simulink model "no1"  (R2024a)
settings: Solver=VariableStepAuto  StartTime=0.0  StopTime=20.0  RelTol=1e-3
values from neighbouring files (symbols this model uses):
  G1_den = [1 0 0]    [BLOCK DIAGRAM NO.1.m]    (also in MALABANAN_MALIBIRAN_NO2_CODE.m; NO1.m)
  G1_num = [0 0 1]    [BLOCK DIAGRAM NO.1.m]    (also in MALABANAN_MALIBIRAN_NO2_CODE.m = [0 1]; NO1.m)
  G2_den = [1 1]    [BLOCK DIAGRAM NO.1.m]    (also in MALABANAN_MALIBIRAN_NO2_CODE.m; NO1.m)
  G2_num = [0 1]    [BLOCK DIAGRAM NO.1.m]    (also in MALABANAN_MALIBIRAN_NO2_CODE.m; NO1.m)
  G2_num_num = [1 2]    [BLOCK DIAGRAM NO.1.m]    (also in NO1.m)
  G2_sum_den = conv(G2_den, G2_num)    [BLOCK DIAGRAM NO.1.m]    (also in NO1.m)
  G3_den = [1 0]    [BLOCK DIAGRAM NO.1.m]    (also in MALABANAN_MALIBIRAN_NO2_CODE.m; NO1.m)
  G3_num = [0 1]    [BLOCK DIAGRAM NO.1.m]    (also in MALABANAN_MALIBIRAN_NO2_CODE.m; NO1.m)
  H1_den = [1 0]    [BLOCK DIAGRAM NO.1.m]    (also in MALABANAN_MALIBIRAN_NO2_CODE.m; NO1.m)
  H1_num = [0 1]    [BLOCK DIAGRAM NO.1.m]    (also in MALABANAN_MALIBIRAN_NO2_CODE.m; NO1.m)
  H2_den = [1 -1]    [BLOCK DIAGRAM NO.1.m]    (also in MALABANAN_MALIBIRAN_NO2_CODE.m; NO1.m)
  H2_num = [0 1]    [BLOCK DIAGRAM NO.1.m]    (also in MALABANAN_MALIBIRAN_NO2_CODE.m; NO1.m)
  H3_den = [1 -2]    [BLOCK DIAGRAM NO.1.m]    (also in MALABANAN_MALIBIRAN_NO2_CODE.m; NO1.m)
  H3_num = [0 1]    [BLOCK DIAGRAM NO.1.m]    (also in MALABANAN_MALIBIRAN_NO2_CODE.m; NO1.m)
  TF2_den = conv(G2_den,TF2_add)    [BLOCK DIAGRAM NO.1.m]    (also in NO1.m)
  TF2_num = conv(GH2_den,GH2_num)    [BLOCK DIAGRAM NO.1.m]    (also in NO1.m)
  TF3_den = conv(G3_den,TF3_add)    [BLOCK DIAGRAM NO.1.m]    (also in NO1.m)
  TF3_num = conv(GH3_den,GH3_num)    [BLOCK DIAGRAM NO.1.m]    (also in NO1.m)
  TF4_den = conv(TF3_den,G2_sum_den)    [BLOCK DIAGRAM NO.1.m]    (also in NO1.m)
  TF4_num = conv(TF3_num,G2_sum_num)    [BLOCK DIAGRAM NO.1.m]    (also in NO1.m)
  TF5_den = conv(TF1_den,TF5_add)    [BLOCK DIAGRAM NO.1.m]    (also in NO1.m)
  TF5_num = conv(TF1_num,TF1H1_den)    [BLOCK DIAGRAM NO.1.m]    (also in NO1.m)
  TF_den = conv(TF5_den,TF4_den)    [BLOCK DIAGRAM NO.1.m]    (also in NO1.m)
  TF_num = conv(TF5_num, TF4_num)    [BLOCK DIAGRAM NO.1.m]    (also in NO1.m)
settings Model: Creator=lenyi  LastModifiedBy=lenyi

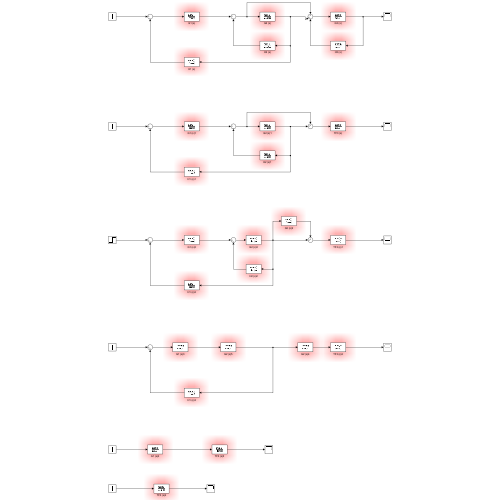
[thumbnail: Simulink's stored preview of the top-level diagram]
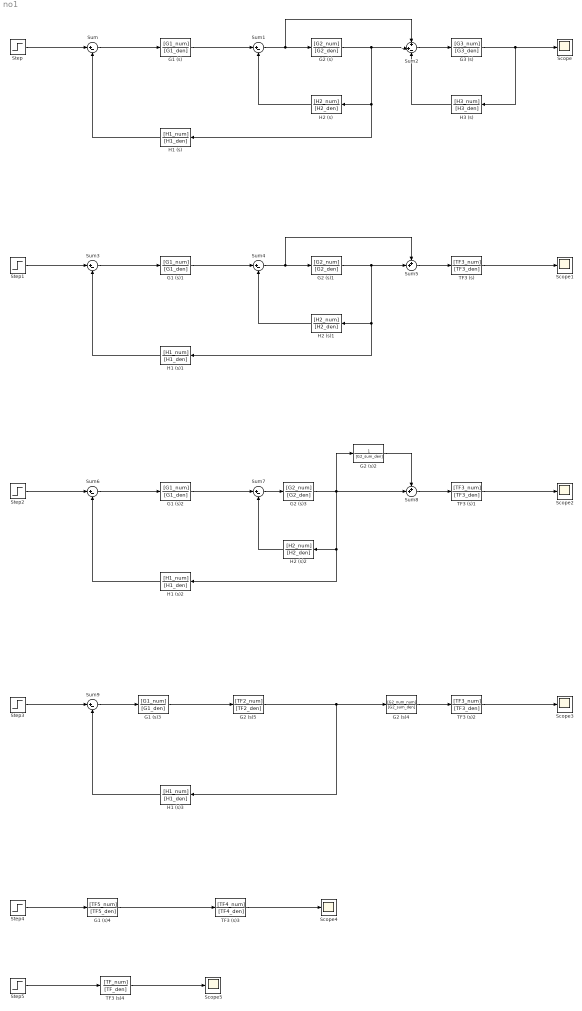
== system no1 ==
  G1 (s){,1..3} (4 alike) : TransferFcn  Numerator=[G1_num]  Denominator=[G1_den]
  G1 (s)4 : TransferFcn  Numerator=[TF5_num]  Denominator=[TF5_den]
  G2 (s) : TransferFcn  Numerator=[G2_num]  Denominator=[G2_den]
  G2 (s)1 : TransferFcn  Numerator=[G2_num]  Denominator=[G2_den]
  G2 (s)2 : TransferFcn  Denominator=[G2_sum_den]
  G2 (s)3 : TransferFcn  Numerator=[G2_num]  Denominator=[G2_den]
  G2 (s)4 : TransferFcn  Numerator=[G2_num_num]  Denominator=[G2_sum_den]
  G2 (s)5 : TransferFcn  Numerator=[TF2_num]  Denominator=[TF2_den]
  G3 (s) : TransferFcn  Numerator=[G3_num]  Denominator=[G3_den]
  H1 (s){,1..3} (4 alike) : TransferFcn  Numerator=[H1_num]  Denominator=[H1_den]
  H2 (s) : TransferFcn  Numerator=[H2_num]  Denominator=[H2_den]
  H2 (s)1 : TransferFcn  Numerator=[H2_num]  Denominator=[H2_den]
  H2 (s)2 : TransferFcn  Numerator=[H2_num]  Denominator=[H2_den]
  H3 (s) : TransferFcn  Numerator=[H3_num]  Denominator=[H3_den]
  Scope{,1..5} (6 alike) : Scope
  Step{,1..5} (6 alike) : Step  SampleTime=0
  Sum{,1,3..4,6..7,9} (7 alike) : Sum  Inputs=|+-
  Sum2 : Sum  Inputs=+|+-
  Sum5 : Sum  Inputs=++|
  Sum8 : Sum  Inputs=++|
  TF3 (s) : TransferFcn  Numerator=[TF3_num]  Denominator=[TF3_den]
  TF3 (s)1 : TransferFcn  Numerator=[TF3_num]  Denominator=[TF3_den]
  TF3 (s)2 : TransferFcn  Numerator=[TF3_num]  Denominator=[TF3_den]
  TF3 (s)3 : TransferFcn  Numerator=[TF4_num]  Denominator=[TF4_den]
  TF3 (s)4 : TransferFcn  Numerator=[TF_num]  Denominator=[TF_den]
  wires:
  Sum2/1 -> G3 (s)/1
  Step/1 -> Sum/1
  Sum/1 -> G1 (s)/1
  H1 (s)/1 -> Sum/2
  G1 (s)/1 -> Sum1/1
  H2 (s)/1 -> Sum1/2
  Sum1/1 -> Sum2/1, G2 (s)/1
  G2 (s)/1 -> H1 (s)/1, H2 (s)/1, Sum2/2
  H3 (s)/1 -> Sum2/3
  G3 (s)/1 -> H3 (s)/1, Scope/1
  TF3 (s)/1 -> Scope1/1
  G2 (s)1/1 -> Sum5/2, H2 (s)1/1, H1 (s)1/1
  Sum4/1 -> G2 (s)1/1, Sum5/1
  H2 (s)1/1 -> Sum4/2
  G1 (s)1/1 -> Sum4/1
  H1 (s)1/1 -> Sum3/2
  Sum3/1 -> G1 (s)1/1
  Step1/1 -> Sum3/1
  Sum5/1 -> TF3 (s)/1
  Sum8/1 -> TF3 (s)1/1
  Step2/1 -> Sum6/1
  Sum6/1 -> G1 (s)2/1
  H1 (s)2/1 -> Sum6/2
  G1 (s)2/1 -> Sum7/1
  H2 (s)2/1 -> Sum7/2
  TF3 (s)1/1 -> Scope2/1
  G2 (s)2/1 -> Sum8/1
  Sum7/1 -> G2 (s)3/1
  G2 (s)3/1 -> H1 (s)2/1, H2 (s)2/1, Sum8/2, G2 (s)2/1
  G2 (s)5/1 -> G2 (s)4/1, H1 (s)3/1
  TF3 (s)2/1 -> Scope3/1
  H1 (s)3/1 -> Sum9/2
  Sum9/1 -> G1 (s)3/1
  Step3/1 -> Sum9/1
  G2 (s)4/1 -> TF3 (s)2/1
  G1 (s)3/1 -> G2 (s)5/1
  TF3 (s)3/1 -> Scope4/1
  Step4/1 -> G1 (s)4/1
  G1 (s)4/1 -> TF3 (s)3/1
  TF3 (s)4/1 -> Scope5/1
  Step5/1 -> TF3 (s)4/1
